simulink model "kurtosis"  (R2012b)
settings: Solver=ode45  StartTime=0.0  StopTime=3171  RelTol=1e-3
libraries: xbsIndex_r4 x3174, casper_library_flow_control x64, casper_library_misc x1, simulink_xsg_bridge x1
(part 1 of 24)
settings Model: Creator=sgowda  LastModifiedBy=sgowda

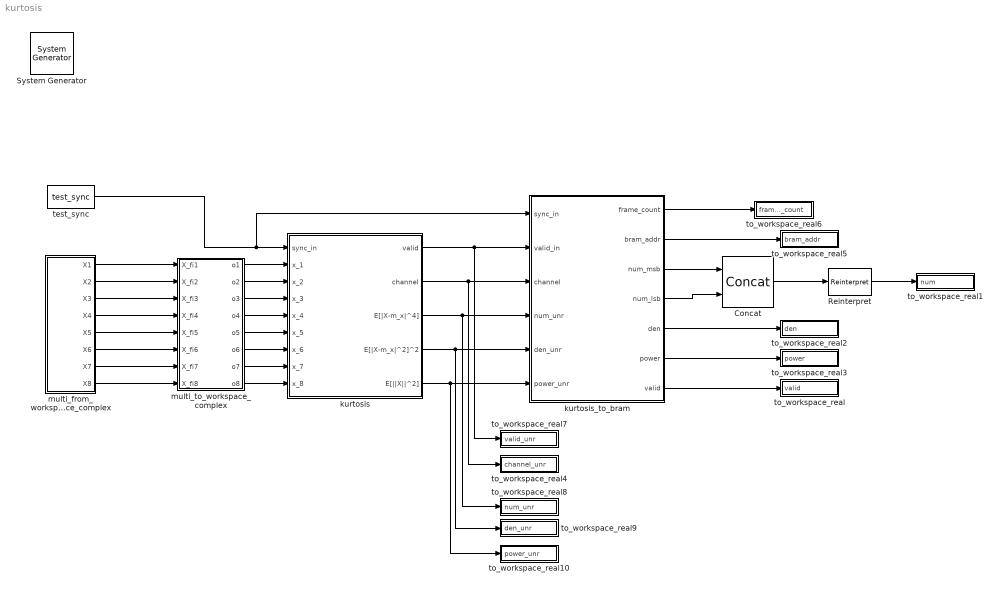
== system kurtosis ==
  " System Generator" : xbsIndex_r4/ System Generator  Tag=genX  xilinxfamily=Kintex7  part=xc7k325t  speed=-3  package=fbg676  synthesis_tool=XST  clock_wrapper=Clock Enables  directory=./netlist  proj_type=Project Navigator  Synth_file=XST Defaults  Impl_file=ISE Defaults  testbench=off  simulink_period=1  sysclk_period=10  dcm_input_clock_period=10  incr_netlist=off  trim_vbits=Everywhere in SubSystem  dbl_ovrd=According to Block Masks  core_generation=According to Block Masks  run_coregen=off  deprecated_control=off  eval_field=0  block_type=sysgen
  Concat : xbsIndex_r4/Concat  num_inputs=2  dbl_ovrd=off  block_type=concat
  Reinterpret : xbsIndex_r4/Reinterpret  force_arith_type=on  arith_type="Signed  (2's comp)"  force_bin_pt=on  bin_pt=84  block_type=reinterpret
  kurtosis : Subsystem
  kurtosis_to_bram : Subsystem
  multi_from_workspace_complex : Subsystem  mask{var_name=X, n_bits=18, bin_pt=17, quantization=Truncate, overflow=Wrap, arith_type=Signed  (2's comp), n_inputs=8}
      mask prompts: var_name "Workspace variable name"; n_bits "# of bits"; bin_pt "Binary Point"; arith_type "Arithmetic type"; n_inputs "# of inputs"
      mask init:
      | config.source = str2func('multi_mat_input_data_cplx_init_xblock');
      |  config.toplevel = gcb();
      |  xBlock(config, {config.toplevel, 'var_name', var_name, ...
      |      'n_bits', n_bits, 'bin_pt', bin_pt, 'quantization', quantization, ...
      |      'overflow', overflow, 'arith_type', arith_type, 'n_inputs', n_inputs});
      mask TypeOptions quantization: Truncate | Round  (unbiased: +/- Inf) | Round  (unbiased: Even Values)
      mask TypeOptions overflow: Wrap | Saturate | Flag as error
      mask TypeOptions arith_type: Signed  (2's comp) | Boolean | Unsigned
  multi_to_workspace_complex : Subsystem  mask{var_name=X_fi, n_bits=18, bin_pt=17, n_inputs=8}
      mask prompts: var_name "Workspace variable name"; n_bits "# of bits"; bin_pt "Binary Point"; n_inputs "# of inputs"
      mask init:
      | config.source = str2func('multi_mat_output_data_cplx_init_xblock');
      | config.toplevel = gcb();
      | xBlock(config, {config.toplevel, 'var_name', var_name, ...
      |     'n_bits', n_bits, 'bin_pt', bin_pt, 'n_inputs', n_inputs});
  test_sync : simulink_xsg_bridge/test_sync
  to_workspace_real : Subsystem  mask{var_name=valid}
      mask prompts: var_name "Workspace variable name"
      mask init:
      | config.source = str2func('mat_output_data_init_xblock');
      | config.toplevel = gcb();
      | xBlock(config, {config.toplevel, 'var_name', var_name});
  to_workspace_real1 : Subsystem  mask{var_name=num}
      mask prompts: var_name "Workspace variable name"
      mask init:
      | config.source = str2func('mat_output_data_init_xblock');
      | config.toplevel = gcb();
      | xBlock(config, {config.toplevel, 'var_name', var_name});
  to_workspace_real10 : Subsystem  mask{var_name=power_unr}
      mask prompts: var_name "Workspace variable name"
      mask init:
      | config.source = str2func('mat_output_data_init_xblock');
      | config.toplevel = gcb();
      | xBlock(config, {config.toplevel, 'var_name', var_name});
  to_workspace_real2 : Subsystem  mask{var_name=den}
      mask prompts: var_name "Workspace variable name"
      mask init:
      | config.source = str2func('mat_output_data_init_xblock');
      | config.toplevel = gcb();
      | xBlock(config, {config.toplevel, 'var_name', var_name});
  to_workspace_real3 : Subsystem  mask{var_name=power}
      mask prompts: var_name "Workspace variable name"
      mask init:
      | config.source = str2func('mat_output_data_init_xblock');
      | config.toplevel = gcb();
      | xBlock(config, {config.toplevel, 'var_name', var_name});
  to_workspace_real4 : Subsystem  mask{var_name=channel_unr}
      mask prompts: var_name "Workspace variable name"
      mask init:
      | config.source = str2func('mat_output_data_init_xblock');
      | config.toplevel = gcb();
      | xBlock(config, {config.toplevel, 'var_name', var_name});
  to_workspace_real5 : Subsystem  mask{var_name=bram_addr}
      mask prompts: var_name "Workspace variable name"
      mask init:
      | config.source = str2func('mat_output_data_init_xblock');
      | config.toplevel = gcb();
      | xBlock(config, {config.toplevel, 'var_name', var_name});
  to_workspace_real6 : Subsystem  mask{var_name=frame_count}
      mask prompts: var_name "Workspace variable name"
      mask init:
      | config.source = str2func('mat_output_data_init_xblock');
      | config.toplevel = gcb();
      | xBlock(config, {config.toplevel, 'var_name', var_name});
  to_workspace_real7 : Subsystem  mask{var_name=valid_unr}
      mask prompts: var_name "Workspace variable name"
      mask init:
      | config.source = str2func('mat_output_data_init_xblock');
      | config.toplevel = gcb();
      | xBlock(config, {config.toplevel, 'var_name', var_name});
  to_workspace_real8 : Subsystem  mask{var_name=num_unr}
      mask prompts: var_name "Workspace variable name"
      mask init:
      | config.source = str2func('mat_output_data_init_xblock');
      | config.toplevel = gcb();
      | xBlock(config, {config.toplevel, 'var_name', var_name});
  to_workspace_real9 : Subsystem  mask{var_name=den_unr}
      mask prompts: var_name "Workspace variable name"
      mask init:
      | config.source = str2func('mat_output_data_init_xblock');
      | config.toplevel = gcb();
      | xBlock(config, {config.toplevel, 'var_name', var_name});
  wires:
  test_sync/1 -> kurtosis_to_bram/1(sync_in), kurtosis/1(sync_in)
  multi_to_workspace_complex/2(o2) -> kurtosis/3(x_2)
  multi_to_workspace_complex/1(o1) -> kurtosis/2(x_1)
  multi_to_workspace_complex/6(o6) -> kurtosis/7(x_6)
  multi_to_workspace_complex/8(o8) -> kurtosis/9(x_8)
  multi_to_workspace_complex/7(o7) -> kurtosis/8(x_7)
  multi_to_workspace_complex/4(o4) -> kurtosis/5(x_4)
  multi_to_workspace_complex/3(o3) -> kurtosis/4(x_3)
  multi_to_workspace_complex/5(o5) -> kurtosis/6(x_5)
  multi_from_workspace_complex/1(X1) -> multi_to_workspace_complex/1(X_fi1)
  multi_from_workspace_complex/8(X8) -> multi_to_workspace_complex/8(X_fi8)
  multi_from_workspace_complex/2(X2) -> multi_to_workspace_complex/2(X_fi2)
  multi_from_workspace_complex/4(X4) -> multi_to_workspace_complex/4(X_fi4)
  multi_from_workspace_complex/7(X7) -> multi_to_workspace_complex/7(X_fi7)
  multi_from_workspace_complex/3(X3) -> multi_to_workspace_complex/3(X_fi3)
  multi_from_workspace_complex/5(X5) -> multi_to_workspace_complex/5(X_fi5)
  multi_from_workspace_complex/6(X6) -> multi_to_workspace_complex/6(X_fi6)
  kurtosis/1(valid) -> to_workspace_real7/1(valid_unr), kurtosis_to_bram/2(valid_in)
  kurtosis/2(channel) -> to_workspace_real4/1(channel_unr), kurtosis_to_bram/3(channel)
  kurtosis/3(E[|X-m_x|^4]) -> kurtosis_to_bram/4(num_unr), to_workspace_real8/1(num_unr)
  kurtosis/4(E[|X-m_x|^2]^2) -> to_workspace_real9/1(den_unr), kurtosis_to_bram/5(den_unr)
  kurtosis_to_bram/1(frame_count) -> to_workspace_real6/1(frame_count)
  kurtosis_to_bram/2(bram_addr) -> to_workspace_real5/1(bram_addr)
  kurtosis_to_bram/7(valid) -> to_workspace_real/1(valid)
  kurtosis_to_bram/5(den) -> to_workspace_real2/1(den)
  kurtosis_to_bram/6(power) -> to_workspace_real3/1(power)
  Reinterpret/1 -> to_workspace_real1/1(num)
  Concat/1 -> Reinterpret/1
  kurtosis_to_bram/3(num_msb) -> Concat/1
  kurtosis_to_bram/4(num_lsb) -> Concat/2
  kurtosis/5(E[||X||^2]) -> to_workspace_real10/1(power_unr), kurtosis_to_bram/6(power_unr)

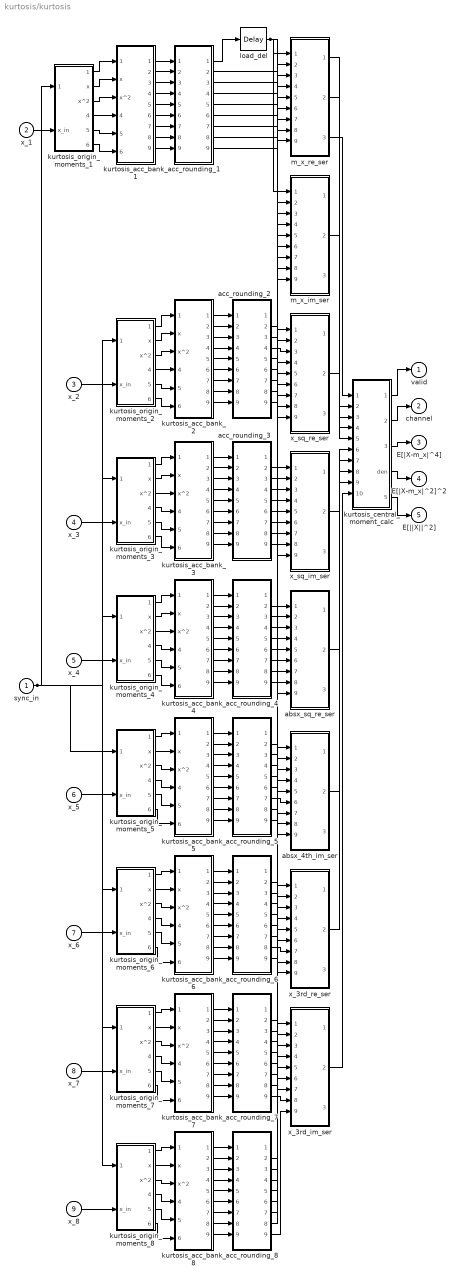
== system kurtosis/kurtosis ==
  sync_in : Inport
  x_1 : Inport  Port=2
  x_2 : Inport  Port=3
  x_3 : Inport  Port=4
  x_4 : Inport  Port=5
  x_5 : Inport  Port=6
  x_6 : Inport  Port=7
  x_7 : Inport  Port=8
  x_8 : Inport  Port=9
  absx_4th_im_ser : Subsystem
  absx_sq_re_ser : Subsystem
  acc_rounding_1 : Subsystem
  acc_rounding_2 : Subsystem
  acc_rounding_3 : Subsystem
  acc_rounding_4 : Subsystem
  acc_rounding_5 : Subsystem
  acc_rounding_6 : Subsystem
  acc_rounding_7 : Subsystem
  acc_rounding_8 : Subsystem
  kurtosis_acc_bank_1 : Subsystem
  kurtosis_acc_bank_2 : Subsystem
  kurtosis_acc_bank_3 : Subsystem
  kurtosis_acc_bank_4 : Subsystem
  kurtosis_acc_bank_5 : Subsystem
  kurtosis_acc_bank_6 : Subsystem
  kurtosis_acc_bank_7 : Subsystem
  kurtosis_acc_bank_8 : Subsystem
  kurtosis_central_moment_calc : Subsystem
  kurtosis_origin_moments_1 : Subsystem
  kurtosis_origin_moments_2 : Subsystem
  kurtosis_origin_moments_3 : Subsystem
  kurtosis_origin_moments_4 : Subsystem
  kurtosis_origin_moments_5 : Subsystem
  kurtosis_origin_moments_6 : Subsystem
  kurtosis_origin_moments_7 : Subsystem
  kurtosis_origin_moments_8 : Subsystem
  load_del : xbsIndex_r4/Delay  rst=off  infoeditControl=Selection of Reset will increase slice count due to use of real FFs and instead of SRLs  en=off  latency=1  dbl_ovrd=off  reg_retiming=off  block_type=delay
  m_x_im_ser : Subsystem
  m_x_re_ser : Subsystem
  x_3rd_im_ser : Subsystem
  x_3rd_re_ser : Subsystem
  x_sq_im_ser : Subsystem
  x_sq_re_ser : Subsystem
  valid : Outport
  channel : Outport  Port=2
  E[|X-m_x|^4] : Outport  Port=3
  E[|X-m_x|^2]^2 : Outport  Port=4
  E[||X||^2] : Outport  Port=5
  wires:
  sync_in/1 -> kurtosis_origin_moments_8/1(sync_in), kurtosis_origin_moments_7/1(sync_in), kurtosis_origin_moments_6/1(sync_in), kurtosis_origin_moments_5/1(sync_in), kurtosis_origin_moments_4/1(sync_in), kurtosis_origin_moments_3/1(sync_in), kurtosis_origin_moments_2/1(sync_in), kurtosis_origin_moments_1/1(sync_in)
  load_del/1 -> x_3rd_im_ser/1(load), x_3rd_re_ser/1(load), absx_4th_im_ser/1(load), absx_sq_re_ser/1(load), x_sq_im_ser/1(load), x_sq_re_ser/1(load), m_x_im_ser/1(load), m_x_re_ser/1(load)
  kurtosis_central_moment_calc/5(power) -> E[||X||^2]/1
  kurtosis_central_moment_calc/4(den) -> E[|X-m_x|^2]^2/1
  kurtosis_central_moment_calc/3(num) -> E[|X-m_x|^4]/1
  kurtosis_central_moment_calc/2(channel) -> channel/1
  kurtosis_central_moment_calc/1(sync_out) -> valid/1
  x_3rd_im_ser/2(ser_data) -> kurtosis_central_moment_calc/10("Im{E[|X|^2X]}")
  x_3rd_re_ser/2(ser_data) -> kurtosis_central_moment_calc/9("Re{E[|X|^2X]}")
  absx_4th_im_ser/2(ser_data) -> kurtosis_central_moment_calc/8(E[||X||^4])
  absx_sq_re_ser/2(ser_data) -> kurtosis_central_moment_calc/7(E[|X|^2])
  x_sq_im_ser/2(ser_data) -> kurtosis_central_moment_calc/6("Im{E[X^2]}")
  x_sq_re_ser/2(ser_data) -> kurtosis_central_moment_calc/5("Re{E[X^2]}")
  m_x_im_ser/2(ser_data) -> kurtosis_central_moment_calc/4("Im{E[X]}")
  m_x_re_ser/2(ser_data) -> kurtosis_central_moment_calc/3("Re{E[X]}")
  m_x_re_ser/1(addr) -> kurtosis_central_moment_calc/2(channel_in)
  m_x_re_ser/3(valid) -> kurtosis_central_moment_calc/1(sync)
  acc_rounding_8/9(X_3rd_acc_im_rounded) -> x_3rd_im_ser/9(din_8)
  acc_rounding_7/9(X_3rd_acc_im_rounded) -> x_3rd_im_ser/8(din_7)
  acc_rounding_6/9(X_3rd_acc_im_rounded) -> x_3rd_im_ser/7(din_6)
  acc_rounding_5/9(X_3rd_acc_im_rounded) -> x_3rd_im_ser/6(din_5)
  acc_rounding_4/9(X_3rd_acc_im_rounded) -> x_3rd_im_ser/5(din_4)
  acc_rounding_3/9(X_3rd_acc_im_rounded) -> x_3rd_im_ser/4(din_3)
  acc_rounding_2/9(X_3rd_acc_im_rounded) -> x_3rd_im_ser/3(din_2)
  acc_rounding_1/9(X_3rd_acc_im_rounded) -> x_3rd_im_ser/2(din_1)
  acc_rounding_8/8(X_3rd_acc_re_rounded) -> x_3rd_re_ser/9(din_8)
  acc_rounding_7/8(X_3rd_acc_re_rounded) -> x_3rd_re_ser/8(din_7)
  acc_rounding_6/8(X_3rd_acc_re_rounded) -> x_3rd_re_ser/7(din_6)
  acc_rounding_5/8(X_3rd_acc_re_rounded) -> x_3rd_re_ser/6(din_5)
  acc_rounding_4/8(X_3rd_acc_re_rounded) -> x_3rd_re_ser/5(din_4)
  acc_rounding_3/8(X_3rd_acc_re_rounded) -> x_3rd_re_ser/4(din_3)
  acc_rounding_2/8(X_3rd_acc_re_rounded) -> x_3rd_re_ser/3(din_2)
  acc_rounding_1/8(X_3rd_acc_re_rounded) -> x_3rd_re_ser/2(din_1)
  acc_rounding_8/7(abs_X_4th_rounded) -> absx_4th_im_ser/9(din_8)
  acc_rounding_7/7(abs_X_4th_rounded) -> absx_4th_im_ser/8(din_7)
  acc_rounding_6/7(abs_X_4th_rounded) -> absx_4th_im_ser/7(din_6)
  acc_rounding_5/7(abs_X_4th_rounded) -> absx_4th_im_ser/6(din_5)
  acc_rounding_4/7(abs_X_4th_rounded) -> absx_4th_im_ser/5(din_4)
  acc_rounding_3/7(abs_X_4th_rounded) -> absx_4th_im_ser/4(din_3)
  acc_rounding_2/7(abs_X_4th_rounded) -> absx_4th_im_ser/3(din_2)
  acc_rounding_1/7(abs_X_4th_rounded) -> absx_4th_im_ser/2(din_1)
  acc_rounding_8/6(abs_X_sq_acc_rounded) -> absx_sq_re_ser/9(din_8)
  acc_rounding_7/6(abs_X_sq_acc_rounded) -> absx_sq_re_ser/8(din_7)
  acc_rounding_6/6(abs_X_sq_acc_rounded) -> absx_sq_re_ser/7(din_6)
  acc_rounding_5/6(abs_X_sq_acc_rounded) -> absx_sq_re_ser/6(din_5)
  acc_rounding_4/6(abs_X_sq_acc_rounded) -> absx_sq_re_ser/5(din_4)
  acc_rounding_3/6(abs_X_sq_acc_rounded) -> absx_sq_re_ser/4(din_3)
  acc_rounding_2/6(abs_X_sq_acc_rounded) -> absx_sq_re_ser/3(din_2)
  acc_rounding_1/6(abs_X_sq_acc_rounded) -> absx_sq_re_ser/2(din_1)
  acc_rounding_8/5(X_sq_acc_im_rounded) -> x_sq_im_ser/9(din_8)
  acc_rounding_7/5(X_sq_acc_im_rounded) -> x_sq_im_ser/8(din_7)
  acc_rounding_6/5(X_sq_acc_im_rounded) -> x_sq_im_ser/7(din_6)
  acc_rounding_5/5(X_sq_acc_im_rounded) -> x_sq_im_ser/6(din_5)
  acc_rounding_4/5(X_sq_acc_im_rounded) -> x_sq_im_ser/5(din_4)
  acc_rounding_3/5(X_sq_acc_im_rounded) -> x_sq_im_ser/4(din_3)
  acc_rounding_2/5(X_sq_acc_im_rounded) -> x_sq_im_ser/3(din_2)
  acc_rounding_1/5(X_sq_acc_im_rounded) -> x_sq_im_ser/2(din_1)
  acc_rounding_8/4(X_sq_acc_re_rounded) -> x_sq_re_ser/9(din_8)
  acc_rounding_7/4(X_sq_acc_re_rounded) -> x_sq_re_ser/8(din_7)
  acc_rounding_6/4(X_sq_acc_re_rounded) -> x_sq_re_ser/7(din_6)
  acc_rounding_5/4(X_sq_acc_re_rounded) -> x_sq_re_ser/6(din_5)
  acc_rounding_4/4(X_sq_acc_re_rounded) -> x_sq_re_ser/5(din_4)
  acc_rounding_3/4(X_sq_acc_re_rounded) -> x_sq_re_ser/4(din_3)
  acc_rounding_2/4(X_sq_acc_re_rounded) -> x_sq_re_ser/3(din_2)
  acc_rounding_1/4(X_sq_acc_re_rounded) -> x_sq_re_ser/2(din_1)
  acc_rounding_8/3(m_x_im_rounded) -> m_x_im_ser/9(din_8)
  acc_rounding_7/3(m_x_im_rounded) -> m_x_im_ser/8(din_7)
  acc_rounding_6/3(m_x_im_rounded) -> m_x_im_ser/7(din_6)
  acc_rounding_5/3(m_x_im_rounded) -> m_x_im_ser/6(din_5)
  acc_rounding_4/3(m_x_im_rounded) -> m_x_im_ser/5(din_4)
  acc_rounding_3/3(m_x_im_rounded) -> m_x_im_ser/4(din_3)
  acc_rounding_2/3(m_x_im_rounded) -> m_x_im_ser/3(din_2)
  acc_rounding_1/3(m_x_im_rounded) -> m_x_im_ser/2(din_1)
  acc_rounding_8/2(m_x_re_rounded) -> m_x_re_ser/9(din_8)
  acc_rounding_7/2(m_x_re_rounded) -> m_x_re_ser/8(din_7)
  acc_rounding_6/2(m_x_re_rounded) -> m_x_re_ser/7(din_6)
  acc_rounding_5/2(m_x_re_rounded) -> m_x_re_ser/6(din_5)
  acc_rounding_4/2(m_x_re_rounded) -> m_x_re_ser/5(din_4)
  acc_rounding_3/2(m_x_re_rounded) -> m_x_re_ser/4(din_3)
  acc_rounding_2/2(m_x_re_rounded) -> m_x_re_ser/3(din_2)
  acc_rounding_1/2(m_x_re_rounded) -> m_x_re_ser/2(din_1)
  acc_rounding_1/1(sync_out) -> load_del/1
  kurtosis_acc_bank_8/9("Im{E[x|x|^2]}") -> acc_rounding_8/9(X_3rd_acc_im)
  kurtosis_acc_bank_8/8("Re{E[x|x|^2]}") -> acc_rounding_8/8(X_3rd_acc_re)
  kurtosis_acc_bank_8/7(E[|x|^4]) -> acc_rounding_8/7(abs_X_4th_acc)
  kurtosis_acc_bank_8/6(E[|x|^2]) -> acc_rounding_8/6(abs_X_sq_acc)
  kurtosis_acc_bank_8/5("Im{E[x^2]}") -> acc_rounding_8/5(X_sq_acc_im)
  kurtosis_acc_bank_8/4("Re{E[x^2]}") -> acc_rounding_8/4(X_sq_acc_re)
  kurtosis_acc_bank_8/3("Im{E[x]}") -> acc_rounding_8/3(x_acc_im)
  kurtosis_acc_bank_8/2("Re{E[x]}") -> acc_rounding_8/2(x_acc_re)
  kurtosis_acc_bank_8/1(sync_out) -> acc_rounding_8/1(sync)
  kurtosis_origin_moments_8/6(x|x|^2) -> kurtosis_acc_bank_8/6(x|x|^2)
  kurtosis_origin_moments_8/5(|x|^4) -> kurtosis_acc_bank_8/5(|x|^4)
  kurtosis_origin_moments_8/4(|x|^2) -> kurtosis_acc_bank_8/4(|x|^2)
  kurtosis_origin_moments_8/3(x^2) -> kurtosis_acc_bank_8/3(x^2)
  kurtosis_origin_moments_8/2(x) -> kurtosis_acc_bank_8/2(x)
  kurtosis_origin_moments_8/1(sync_out) -> kurtosis_acc_bank_8/1(sync)
  x_8/1 -> kurtosis_origin_moments_8/2(x_in)
  kurtosis_acc_bank_7/9("Im{E[x|x|^2]}") -> acc_rounding_7/9(X_3rd_acc_im)
  kurtosis_acc_bank_7/8("Re{E[x|x|^2]}") -> acc_rounding_7/8(X_3rd_acc_re)
  kurtosis_acc_bank_7/7(E[|x|^4]) -> acc_rounding_7/7(abs_X_4th_acc)
  kurtosis_acc_bank_7/6(E[|x|^2]) -> acc_rounding_7/6(abs_X_sq_acc)
  kurtosis_acc_bank_7/5("Im{E[x^2]}") -> acc_rounding_7/5(X_sq_acc_im)
  kurtosis_acc_bank_7/4("Re{E[x^2]}") -> acc_rounding_7/4(X_sq_acc_re)
  kurtosis_acc_bank_7/3("Im{E[x]}") -> acc_rounding_7/3(x_acc_im)
  kurtosis_acc_bank_7/2("Re{E[x]}") -> acc_rounding_7/2(x_acc_re)
  kurtosis_acc_bank_7/1(sync_out) -> acc_rounding_7/1(sync)
  kurtosis_origin_moments_7/6(x|x|^2) -> kurtosis_acc_bank_7/6(x|x|^2)
  kurtosis_origin_moments_7/5(|x|^4) -> kurtosis_acc_bank_7/5(|x|^4)
  kurtosis_origin_moments_7/4(|x|^2) -> kurtosis_acc_bank_7/4(|x|^2)
  kurtosis_origin_moments_7/3(x^2) -> kurtosis_acc_bank_7/3(x^2)
  kurtosis_origin_moments_7/2(x) -> kurtosis_acc_bank_7/2(x)
  kurtosis_origin_moments_7/1(sync_out) -> kurtosis_acc_bank_7/1(sync)
  x_7/1 -> kurtosis_origin_moments_7/2(x_in)
  kurtosis_acc_bank_6/9("Im{E[x|x|^2]}") -> acc_rounding_6/9(X_3rd_acc_im)
  kurtosis_acc_bank_6/8("Re{E[x|x|^2]}") -> acc_rounding_6/8(X_3rd_acc_re)
  kurtosis_acc_bank_6/7(E[|x|^4]) -> acc_rounding_6/7(abs_X_4th_acc)
  kurtosis_acc_bank_6/6(E[|x|^2]) -> acc_rounding_6/6(abs_X_sq_acc)
  kurtosis_acc_bank_6/5("Im{E[x^2]}") -> acc_rounding_6/5(X_sq_acc_im)
  kurtosis_acc_bank_6/4("Re{E[x^2]}") -> acc_rounding_6/4(X_sq_acc_re)
  kurtosis_acc_bank_6/3("Im{E[x]}") -> acc_rounding_6/3(x_acc_im)
  kurtosis_acc_bank_6/2("Re{E[x]}") -> acc_rounding_6/2(x_acc_re)
  kurtosis_acc_bank_6/1(sync_out) -> acc_rounding_6/1(sync)
  kurtosis_origin_moments_6/6(x|x|^2) -> kurtosis_acc_bank_6/6(x|x|^2)
  kurtosis_origin_moments_6/5(|x|^4) -> kurtosis_acc_bank_6/5(|x|^4)
  kurtosis_origin_moments_6/4(|x|^2) -> kurtosis_acc_bank_6/4(|x|^2)
  kurtosis_origin_moments_6/3(x^2) -> kurtosis_acc_bank_6/3(x^2)
  kurtosis_origin_moments_6/2(x) -> kurtosis_acc_bank_6/2(x)
  kurtosis_origin_moments_6/1(sync_out) -> kurtosis_acc_bank_6/1(sync)
  x_6/1 -> kurtosis_origin_moments_6/2(x_in)
  kurtosis_acc_bank_5/9("Im{E[x|x|^2]}") -> acc_rounding_5/9(X_3rd_acc_im)
  kurtosis_acc_bank_5/8("Re{E[x|x|^2]}") -> acc_rounding_5/8(X_3rd_acc_re)
  kurtosis_acc_bank_5/7(E[|x|^4]) -> acc_rounding_5/7(abs_X_4th_acc)
  kurtosis_acc_bank_5/6(E[|x|^2]) -> acc_rounding_5/6(abs_X_sq_acc)
  kurtosis_acc_bank_5/5("Im{E[x^2]}") -> acc_rounding_5/5(X_sq_acc_im)
  kurtosis_acc_bank_5/4("Re{E[x^2]}") -> acc_rounding_5/4(X_sq_acc_re)
  kurtosis_acc_bank_5/3("Im{E[x]}") -> acc_rounding_5/3(x_acc_im)
  kurtosis_acc_bank_5/2("Re{E[x]}") -> acc_rounding_5/2(x_acc_re)
  kurtosis_acc_bank_5/1(sync_out) -> acc_rounding_5/1(sync)
  kurtosis_origin_moments_5/6(x|x|^2) -> kurtosis_acc_bank_5/6(x|x|^2)
  kurtosis_origin_moments_5/5(|x|^4) -> kurtosis_acc_bank_5/5(|x|^4)
  kurtosis_origin_moments_5/4(|x|^2) -> kurtosis_acc_bank_5/4(|x|^2)
  kurtosis_origin_moments_5/3(x^2) -> kurtosis_acc_bank_5/3(x^2)
  kurtosis_origin_moments_5/2(x) -> kurtosis_acc_bank_5/2(x)
  kurtosis_origin_moments_5/1(sync_out) -> kurtosis_acc_bank_5/1(sync)
  x_5/1 -> kurtosis_origin_moments_5/2(x_in)
  kurtosis_acc_bank_4/9("Im{E[x|x|^2]}") -> acc_rounding_4/9(X_3rd_acc_im)
  kurtosis_acc_bank_4/8("Re{E[x|x|^2]}") -> acc_rounding_4/8(X_3rd_acc_re)
  kurtosis_acc_bank_4/7(E[|x|^4]) -> acc_rounding_4/7(abs_X_4th_acc)
  kurtosis_acc_bank_4/6(E[|x|^2]) -> acc_rounding_4/6(abs_X_sq_acc)
  kurtosis_acc_bank_4/5("Im{E[x^2]}") -> acc_rounding_4/5(X_sq_acc_im)
  kurtosis_acc_bank_4/4("Re{E[x^2]}") -> acc_rounding_4/4(X_sq_acc_re)
  kurtosis_acc_bank_4/3("Im{E[x]}") -> acc_rounding_4/3(x_acc_im)
  kurtosis_acc_bank_4/2("Re{E[x]}") -> acc_rounding_4/2(x_acc_re)
  kurtosis_acc_bank_4/1(sync_out) -> acc_rounding_4/1(sync)
  kurtosis_origin_moments_4/6(x|x|^2) -> kurtosis_acc_bank_4/6(x|x|^2)
  kurtosis_origin_moments_4/5(|x|^4) -> kurtosis_acc_bank_4/5(|x|^4)
  kurtosis_origin_moments_4/4(|x|^2) -> kurtosis_acc_bank_4/4(|x|^2)
  kurtosis_origin_moments_4/3(x^2) -> kurtosis_acc_bank_4/3(x^2)
  kurtosis_origin_moments_4/2(x) -> kurtosis_acc_bank_4/2(x)
  kurtosis_origin_moments_4/1(sync_out) -> kurtosis_acc_bank_4/1(sync)
  x_4/1 -> kurtosis_origin_moments_4/2(x_in)
  kurtosis_acc_bank_3/9("Im{E[x|x|^2]}") -> acc_rounding_3/9(X_3rd_acc_im)
  kurtosis_acc_bank_3/8("Re{E[x|x|^2]}") -> acc_rounding_3/8(X_3rd_acc_re)
  kurtosis_acc_bank_3/7(E[|x|^4]) -> acc_rounding_3/7(abs_X_4th_acc)
  kurtosis_acc_bank_3/6(E[|x|^2]) -> acc_rounding_3/6(abs_X_sq_acc)
  kurtosis_acc_bank_3/5("Im{E[x^2]}") -> acc_rounding_3/5(X_sq_acc_im)
  kurtosis_acc_bank_3/4("Re{E[x^2]}") -> acc_rounding_3/4(X_sq_acc_re)
  kurtosis_acc_bank_3/3("Im{E[x]}") -> acc_rounding_3/3(x_acc_im)
  kurtosis_acc_bank_3/2("Re{E[x]}") -> acc_rounding_3/2(x_acc_re)
  kurtosis_acc_bank_3/1(sync_out) -> acc_rounding_3/1(sync)
  kurtosis_origin_moments_3/6(x|x|^2) -> kurtosis_acc_bank_3/6(x|x|^2)
  kurtosis_origin_moments_3/5(|x|^4) -> kurtosis_acc_bank_3/5(|x|^4)
  kurtosis_origin_moments_3/4(|x|^2) -> kurtosis_acc_bank_3/4(|x|^2)
  kurtosis_origin_moments_3/3(x^2) -> kurtosis_acc_bank_3/3(x^2)
  kurtosis_origin_moments_3/2(x) -> kurtosis_acc_bank_3/2(x)
  kurtosis_origin_moments_3/1(sync_out) -> kurtosis_acc_bank_3/1(sync)
  x_3/1 -> kurtosis_origin_moments_3/2(x_in)
  kurtosis_acc_bank_2/9("Im{E[x|x|^2]}") -> acc_rounding_2/9(X_3rd_acc_im)
  kurtosis_acc_bank_2/8("Re{E[x|x|^2]}") -> acc_rounding_2/8(X_3rd_acc_re)
  kurtosis_acc_bank_2/7(E[|x|^4]) -> acc_rounding_2/7(abs_X_4th_acc)
  kurtosis_acc_bank_2/6(E[|x|^2]) -> acc_rounding_2/6(abs_X_sq_acc)
  kurtosis_acc_bank_2/5("Im{E[x^2]}") -> acc_rounding_2/5(X_sq_acc_im)
  kurtosis_acc_bank_2/4("Re{E[x^2]}") -> acc_rounding_2/4(X_sq_acc_re)
  kurtosis_acc_bank_2/3("Im{E[x]}") -> acc_rounding_2/3(x_acc_im)
  kurtosis_acc_bank_2/2("Re{E[x]}") -> acc_rounding_2/2(x_acc_re)
  kurtosis_acc_bank_2/1(sync_out) -> acc_rounding_2/1(sync)
  kurtosis_origin_moments_2/6(x|x|^2) -> kurtosis_acc_bank_2/6(x|x|^2)
  kurtosis_origin_moments_2/5(|x|^4) -> kurtosis_acc_bank_2/5(|x|^4)
  kurtosis_origin_moments_2/4(|x|^2) -> kurtosis_acc_bank_2/4(|x|^2)
  kurtosis_origin_moments_2/3(x^2) -> kurtosis_acc_bank_2/3(x^2)
  kurtosis_origin_moments_2/2(x) -> kurtosis_acc_bank_2/2(x)
  kurtosis_origin_moments_2/1(sync_out) -> kurtosis_acc_bank_2/1(sync)
  x_2/1 -> kurtosis_origin_moments_2/2(x_in)
  kurtosis_acc_bank_1/9("Im{E[x|x|^2]}") -> acc_rounding_1/9(X_3rd_acc_im)
  kurtosis_acc_bank_1/8("Re{E[x|x|^2]}") -> acc_rounding_1/8(X_3rd_acc_re)
  kurtosis_acc_bank_1/7(E[|x|^4]) -> acc_rounding_1/7(abs_X_4th_acc)
  kurtosis_acc_bank_1/6(E[|x|^2]) -> acc_rounding_1/6(abs_X_sq_acc)
  kurtosis_acc_bank_1/5("Im{E[x^2]}") -> acc_rounding_1/5(X_sq_acc_im)
  kurtosis_acc_bank_1/4("Re{E[x^2]}") -> acc_rounding_1/4(X_sq_acc_re)
  kurtosis_acc_bank_1/3("Im{E[x]}") -> acc_rounding_1/3(x_acc_im)
  kurtosis_acc_bank_1/2("Re{E[x]}") -> acc_rounding_1/2(x_acc_re)
  kurtosis_acc_bank_1/1(sync_out) -> acc_rounding_1/1(sync)
  kurtosis_origin_moments_1/6(x|x|^2) -> kurtosis_acc_bank_1/6(x|x|^2)
  kurtosis_origin_moments_1/5(|x|^4) -> kurtosis_acc_bank_1/5(|x|^4)
  kurtosis_origin_moments_1/4(|x|^2) -> kurtosis_acc_bank_1/4(|x|^2)
  kurtosis_origin_moments_1/3(x^2) -> kurtosis_acc_bank_1/3(x^2)
  kurtosis_origin_moments_1/2(x) -> kurtosis_acc_bank_1/2(x)
  kurtosis_origin_moments_1/1(sync_out) -> kurtosis_acc_bank_1/1(sync)
  x_1/1 -> kurtosis_origin_moments_1/2(x_in)

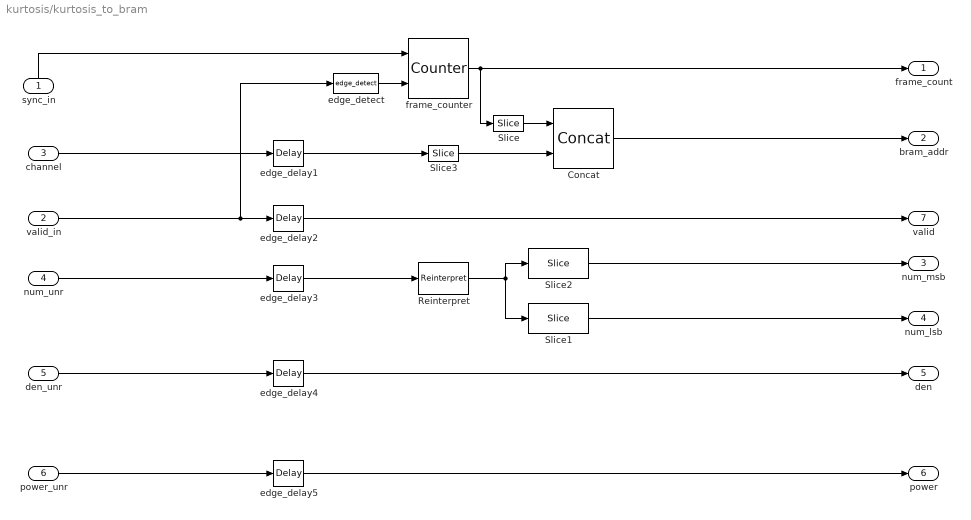
== system kurtosis/kurtosis_to_bram ==
  sync_in : Inport
  valid_in : Inport  Port=2
  channel : Inport  Port=3
  num_unr : Inport  Port=4
  den_unr : Inport  Port=5
  power_unr : Inport  Port=6
  Concat : xbsIndex_r4/Concat  num_inputs=2  dbl_ovrd=off  block_type=concat
  Reinterpret : xbsIndex_r4/Reinterpret  force_arith_type=on  arith_type=Unsigned  force_bin_pt=on  bin_pt=0  block_type=reinterpret
  Slice : xbsIndex_r4/Slice  nbits=7  boolean_output=off  mode=Lower Bit Location + Width  bit1=0  base1=MSB of Input  bit0=0  base0=LSB of Input  dbl_ovrd=off  block_type=slice
  Slice1 : xbsIndex_r4/Slice  nbits=64  boolean_output=off  mode=Lower Bit Location + Width  bit1=0  base1=MSB of Input  bit0=0  base0=LSB of Input  dbl_ovrd=off  block_type=slice
  Slice2 : xbsIndex_r4/Slice  nbits=32  boolean_output=off  mode=Lower Bit Location + Width  bit1=0  base1=MSB of Input  bit0=64  base0=LSB of Input  dbl_ovrd=off  block_type=slice
  Slice3 : xbsIndex_r4/Slice  nbits=3  boolean_output=off  mode=Lower Bit Location + Width  bit1=0  base1=MSB of Input  bit0=0  base0=LSB of Input  dbl_ovrd=off  block_type=slice
  edge_delay{1..5} (5 alike) : xbsIndex_r4/Delay  rst=off  infoeditControl=Selection of Reset will increase slice count due to use of real FFs and instead of SRLs  en=off  latency=1  dbl_ovrd=off  reg_retiming=off  block_type=delay
  edge_detect : casper_library_misc/edge_detect  edge=Rising  polarity=Active High  x_in=[0 0.08 0.08 0.16 0.16 0.24 0.24 0.32 0.32 0.4]  y_in="[-1 -1  1  1  1  1  1  1  1  1]"  x_out=[0.6 0.68 0.68 0.76 0.76 0.84 0.84 0.92 0.92 1]  y_out="[-1 -1  1  1 -1 -1 -1 -1 -1 -1]"
  frame_counter : xbsIndex_r4/Counter  cnt_type=Free Running  cnt_to=Inf  operation=Up  start_count=0  cnt_by_val=1  arith_type=Unsigned  n_bits=48  bin_pt=0  load_pin=off  rst=on  en=on  explicit_period=on  period=1  dbl_ovrd=off  use_behavioral_HDL=off  implementation=DSP48  block_type=counter
  frame_count : Outport
  bram_addr : Outport  Port=2
  num_msb : Outport  Port=3
  num_lsb : Outport  Port=4
  den : Outport  Port=5
  power : Outport  Port=6
  valid : Outport  Port=7
  wires:
  Slice3/1 -> Concat/2
  Slice/1 -> Concat/1
  valid_in/1 -> edge_detect/1, edge_delay2/1
  edge_delay1/1 -> Slice3/1
  Concat/1 -> bram_addr/1
  edge_detect/1 -> frame_counter/2
  edge_delay5/1 -> power/1
  edge_delay4/1 -> den/1
  edge_delay3/1 -> Reinterpret/1
  frame_counter/1 -> frame_count/1, Slice/1
  channel/1 -> edge_delay1/1
  edge_delay2/1 -> valid/1
  Reinterpret/1 -> Slice1/1, Slice2/1
  sync_in/1 -> frame_counter/1
  Slice2/1 -> num_msb/1
  Slice1/1 -> num_lsb/1
  num_unr/1 -> edge_delay3/1
  den_unr/1 -> edge_delay4/1
  power_unr/1 -> edge_delay5/1

== system kurtosis/multi_from_workspace_complex ==
  from_workspace_cplx_1 : Subsystem
  from_workspace_cplx_2 : Subsystem
  from_workspace_cplx_3 : Subsystem
  from_workspace_cplx_4 : Subsystem
  from_workspace_cplx_5 : Subsystem
  from_workspace_cplx_6 : Subsystem
  from_workspace_cplx_7 : Subsystem
  from_workspace_cplx_8 : Subsystem
  X1 : Outport
  X2 : Outport  Port=2
  X3 : Outport  Port=3
  X4 : Outport  Port=4
  X5 : Outport  Port=5
  X6 : Outport  Port=6
  X7 : Outport  Port=7
  X8 : Outport  Port=8
  wires:
  from_workspace_cplx_8/1(X8) -> X8/1
  from_workspace_cplx_7/1(X7) -> X7/1
  from_workspace_cplx_6/1(X6) -> X6/1
  from_workspace_cplx_5/1(X5) -> X5/1
  from_workspace_cplx_4/1(X4) -> X4/1
  from_workspace_cplx_3/1(X3) -> X3/1
  from_workspace_cplx_2/1(X2) -> X2/1
  from_workspace_cplx_1/1(X1) -> X1/1

== system kurtosis/multi_to_workspace_complex ==
  X_fi1 : Inport
  X_fi2 : Inport  Port=2
  X_fi3 : Inport  Port=3
  X_fi4 : Inport  Port=4
  X_fi5 : Inport  Port=5
  X_fi6 : Inport  Port=6
  X_fi7 : Inport  Port=7
  X_fi8 : Inport  Port=8
  to_workspace_cplx_1 : Subsystem
  to_workspace_cplx_2 : Subsystem
  to_workspace_cplx_3 : Subsystem
  to_workspace_cplx_4 : Subsystem
  to_workspace_cplx_5 : Subsystem
  to_workspace_cplx_6 : Subsystem
  to_workspace_cplx_7 : Subsystem
  to_workspace_cplx_8 : Subsystem
  o1 : Outport
  o2 : Outport  Port=2
  o3 : Outport  Port=3
  o4 : Outport  Port=4
  o5 : Outport  Port=5
  o6 : Outport  Port=6
  o7 : Outport  Port=7
  o8 : Outport  Port=8
  wires:
  to_workspace_cplx_8/1(_o) -> o8/1
  X_fi8/1 -> to_workspace_cplx_8/1(X_fi8)
  to_workspace_cplx_7/1(_o) -> o7/1
  X_fi7/1 -> to_workspace_cplx_7/1(X_fi7)
  to_workspace_cplx_6/1(_o) -> o6/1
  X_fi6/1 -> to_workspace_cplx_6/1(X_fi6)
  to_workspace_cplx_5/1(_o) -> o5/1
  X_fi5/1 -> to_workspace_cplx_5/1(X_fi5)
  to_workspace_cplx_4/1(_o) -> o4/1
  X_fi4/1 -> to_workspace_cplx_4/1(X_fi4)
  to_workspace_cplx_3/1(_o) -> o3/1
  X_fi3/1 -> to_workspace_cplx_3/1(X_fi3)
  to_workspace_cplx_2/1(_o) -> o2/1
  X_fi2/1 -> to_workspace_cplx_2/1(X_fi2)
  to_workspace_cplx_1/1(_o) -> o1/1
  X_fi1/1 -> to_workspace_cplx_1/1(X_fi1)

== system kurtosis/to_workspace_real ==
  valid : Inport
  gateway : xbsIndex_r4/Gateway Out  inherit_from_input=on  hdl_port=off  timing_constraint=None  locs_specified=off  LOCs={}  UseAsDAC=off  DACChannel='1'  block_type=gatewayout
  workspace_input : ToWorkspace  VariableName=valid  SampleTime=-1
  wires:
  gateway/1 -> workspace_input/1
  valid/1 -> gateway/1

== system kurtosis/to_workspace_real1 ==
  num : Inport
  gateway : xbsIndex_r4/Gateway Out  inherit_from_input=on  hdl_port=off  timing_constraint=None  locs_specified=off  LOCs={}  UseAsDAC=off  DACChannel='1'  block_type=gatewayout
  workspace_input : ToWorkspace  VariableName=num  SampleTime=-1
  wires:
  gateway/1 -> workspace_input/1
  num/1 -> gateway/1

== system kurtosis/to_workspace_real10 ==
  power_unr : Inport
  gateway : xbsIndex_r4/Gateway Out  inherit_from_input=on  hdl_port=off  timing_constraint=None  locs_specified=off  LOCs={}  UseAsDAC=off  DACChannel='1'  block_type=gatewayout
  workspace_input : ToWorkspace  VariableName=power_unr  SampleTime=-1
  wires:
  gateway/1 -> workspace_input/1
  power_unr/1 -> gateway/1

== system kurtosis/to_workspace_real2 ==
  den : Inport
  gateway : xbsIndex_r4/Gateway Out  inherit_from_input=on  hdl_port=off  timing_constraint=None  locs_specified=off  LOCs={}  UseAsDAC=off  DACChannel='1'  block_type=gatewayout
  workspace_input : ToWorkspace  VariableName=den  SampleTime=-1
  wires:
  gateway/1 -> workspace_input/1
  den/1 -> gateway/1

== system kurtosis/to_workspace_real3 ==
  power : Inport
  gateway : xbsIndex_r4/Gateway Out  inherit_from_input=on  hdl_port=off  timing_constraint=None  locs_specified=off  LOCs={}  UseAsDAC=off  DACChannel='1'  block_type=gatewayout
  workspace_input : ToWorkspace  VariableName=power  SampleTime=-1
  wires:
  gateway/1 -> workspace_input/1
  power/1 -> gateway/1

== system kurtosis/to_workspace_real4 ==
  channel_unr : Inport
  gateway : xbsIndex_r4/Gateway Out  inherit_from_input=on  hdl_port=off  timing_constraint=None  locs_specified=off  LOCs={}  UseAsDAC=off  DACChannel='1'  block_type=gatewayout
  workspace_input : ToWorkspace  VariableName=channel_unr  SampleTime=-1
  wires:
  gateway/1 -> workspace_input/1
  channel_unr/1 -> gateway/1

== system kurtosis/to_workspace_real5 ==
  bram_addr : Inport
  gateway : xbsIndex_r4/Gateway Out  inherit_from_input=on  hdl_port=off  timing_constraint=None  locs_specified=off  LOCs={}  UseAsDAC=off  DACChannel='1'  block_type=gatewayout
  workspace_input : ToWorkspace  VariableName=bram_addr  SampleTime=-1
  wires:
  gateway/1 -> workspace_input/1
  bram_addr/1 -> gateway/1

== system kurtosis/to_workspace_real6 ==
  frame_count : Inport
  gateway : xbsIndex_r4/Gateway Out  inherit_from_input=on  hdl_port=off  timing_constraint=None  locs_specified=off  LOCs={}  UseAsDAC=off  DACChannel='1'  block_type=gatewayout
  workspace_input : ToWorkspace  VariableName=frame_count  SampleTime=-1
  wires:
  gateway/1 -> workspace_input/1
  frame_count/1 -> gateway/1

== system kurtosis/to_workspace_real7 ==
  valid_unr : Inport
  gateway : xbsIndex_r4/Gateway Out  inherit_from_input=on  hdl_port=off  timing_constraint=None  locs_specified=off  LOCs={}  UseAsDAC=off  DACChannel='1'  block_type=gatewayout
  workspace_input : ToWorkspace  VariableName=valid_unr  SampleTime=-1
  wires:
  gateway/1 -> workspace_input/1
  valid_unr/1 -> gateway/1

== system kurtosis/to_workspace_real8 ==
  num_unr : Inport
  gateway : xbsIndex_r4/Gateway Out  inherit_from_input=on  hdl_port=off  timing_constraint=None  locs_specified=off  LOCs={}  UseAsDAC=off  DACChannel='1'  block_type=gatewayout
  workspace_input : ToWorkspace  VariableName=num_unr  SampleTime=-1
  wires:
  gateway/1 -> workspace_input/1
  num_unr/1 -> gateway/1

== system kurtosis/to_workspace_real9 ==
  den_unr : Inport
  gateway : xbsIndex_r4/Gateway Out  inherit_from_input=on  hdl_port=off  timing_constraint=None  locs_specified=off  LOCs={}  UseAsDAC=off  DACChannel='1'  block_type=gatewayout
  workspace_input : ToWorkspace  VariableName=den_unr  SampleTime=-1
  wires:
  gateway/1 -> workspace_input/1
  den_unr/1 -> gateway/1

== system kurtosis/kurtosis/absx_4th_im_ser ==
  load : Inport
  din_1 : Inport  Port=2
  din_2 : Inport  Port=3
  din_3 : Inport  Port=4
  din_4 : Inport  Port=5
  din_5 : Inport  Port=6
  din_6 : Inport  Port=7
  din_7 : Inport  Port=8
  din_8 : Inport  Port=9
  addr_counter : xbsIndex_r4/Counter  cnt_type=Free Running  cnt_to=Inf  operation=Up  start_count=0  cnt_by_val=1  arith_type=Unsigned  n_bits=4  bin_pt=0  load_pin=off  rst=on  en=off  explicit_period=on  period=1  dbl_ovrd=off  use_behavioral_HDL=off  implementation=Fabric  block_type=counter
  addr_del : xbsIndex_r4/Delay  rst=off  infoeditControl=Selection of Reset will increase slice count due to use of real FFs and instead of SRLs  en=off  latency=1  dbl_ovrd=off  reg_retiming=off  block_type=delay
  par_to_ser : Subsystem  AncestorBlock=casper_library_flow_control/parallel_to_serial_converter  mask(parallel_to_serial_converter){pin_width=672, sout_width=84}
      mask prompts: pin_width "Parallel Input Width"; sout_width "Serial Output Width"
      mask help:
      | This block takes as input a parallel bus of specified width.
      | When the load signal 'ld' is asserted, this data is broken into
      | pieces of width specified by the serial output width and
      | stored into different registers chained to form a shift register.
      | If the 'shift' input is subsequently asserted, the shift register
      | returns as output a new piece of data of width sout_width.  This data
      | is the next least significant piece of the original bus.  The converter
      | serializes SMALL ENDIAN.
      |
      | Note that the load operation automatically loads the least significant
      | bits into the register closest to the output, so the first 'shift'
      | assertion changes the data output from bits [sout_width-1:0] to
      | bits [2*sout_width-1:sout_width].
      mask init:
      | parallel_to_serial_converter_init(gcb, ...
      |     'pin_width', pin_width, ...
      |     'sout_width', sout_width);
  pin_concat : Subsystem
  pulse_ext : Subsystem
  reinterp : xbsIndex_r4/Reinterpret  force_arith_type=on  arith_type="Signed  (2's comp)"  force_bin_pt=on  bin_pt=68  block_type=reinterpret
  addr : Outport
  ser_data : Outport  Port=2
  valid : Outport  Port=3
  wires:
  load/1 -> addr_counter/1, par_to_ser/2(ld), pulse_ext/1(ld)
  pulse_ext/1(shift) -> par_to_ser/3(shift), valid/1  "shift"
  addr_del/1 -> addr/1
  addr_counter/1 -> addr_del/1
  reinterp/1 -> ser_data/1
  par_to_ser/1(sout) -> reinterp/1  "sout"
  pin_concat/1(out) -> par_to_ser/1(pin)
  din_8/1 -> pin_concat/8(in7)
  din_7/1 -> pin_concat/7(in6)
  din_6/1 -> pin_concat/6(in5)
  din_5/1 -> pin_concat/5(in4)
  din_4/1 -> pin_concat/4(in3)
  din_3/1 -> pin_concat/3(in2)
  din_2/1 -> pin_concat/2(in1)
  din_1/1 -> pin_concat/1(in0)

== system kurtosis/kurtosis/absx_sq_re_ser ==
  load : Inport
  din_1 : Inport  Port=2
  din_2 : Inport  Port=3
  din_3 : Inport  Port=4
  din_4 : Inport  Port=5
  din_5 : Inport  Port=6
  din_6 : Inport  Port=7
  din_7 : Inport  Port=8
  din_8 : Inport  Port=9
  addr_counter : xbsIndex_r4/Counter  cnt_type=Free Running  cnt_to=Inf  operation=Up  start_count=0  cnt_by_val=1  arith_type=Unsigned  n_bits=4  bin_pt=0  load_pin=off  rst=on  en=off  explicit_period=on  period=1  dbl_ovrd=off  use_behavioral_HDL=off  implementation=Fabric  block_type=counter
  addr_del : xbsIndex_r4/Delay  rst=off  infoeditControl=Selection of Reset will increase slice count due to use of real FFs and instead of SRLs  en=off  latency=1  dbl_ovrd=off  reg_retiming=off  block_type=delay
  par_to_ser : Subsystem  AncestorBlock=casper_library_flow_control/parallel_to_serial_converter  mask(parallel_to_serial_converter){pin_width=280, sout_width=35}
      mask prompts: pin_width "Parallel Input Width"; sout_width "Serial Output Width"
      mask help:
      | This block takes as input a parallel bus of specified width.
      | When the load signal 'ld' is asserted, this data is broken into
      | pieces of width specified by the serial output width and
      | stored into different registers chained to form a shift register.
      | If the 'shift' input is subsequently asserted, the shift register
      | returns as output a new piece of data of width sout_width.  This data
      | is the next least significant piece of the original bus.  The converter
      | serializes SMALL ENDIAN.
      |
      | Note that the load operation automatically loads the least significant
      | bits into the register closest to the output, so the first 'shift'
      | assertion changes the data output from bits [sout_width-1:0] to
      | bits [2*sout_width-1:sout_width].
      mask init:
      | parallel_to_serial_converter_init(gcb, ...
      |     'pin_width', pin_width, ...
      |     'sout_width', sout_width);
  pin_concat : Subsystem
  pulse_ext : Subsystem
  reinterp : xbsIndex_r4/Reinterpret  force_arith_type=on  arith_type="Signed  (2's comp)"  force_bin_pt=on  bin_pt=22  block_type=reinterpret
  addr : Outport
  ser_data : Outport  Port=2
  valid : Outport  Port=3
  wires:
  load/1 -> addr_counter/1, par_to_ser/2(ld), pulse_ext/1(ld)
  pulse_ext/1(shift) -> par_to_ser/3(shift), valid/1  "shift"
  addr_del/1 -> addr/1
  addr_counter/1 -> addr_del/1
  reinterp/1 -> ser_data/1
  par_to_ser/1(sout) -> reinterp/1  "sout"
  pin_concat/1(out) -> par_to_ser/1(pin)
  din_8/1 -> pin_concat/8(in7)
  din_7/1 -> pin_concat/7(in6)
  din_6/1 -> pin_concat/6(in5)
  din_5/1 -> pin_concat/5(in4)
  din_4/1 -> pin_concat/4(in3)
  din_3/1 -> pin_concat/3(in2)
  din_2/1 -> pin_concat/2(in1)
  din_1/1 -> pin_concat/1(in0)

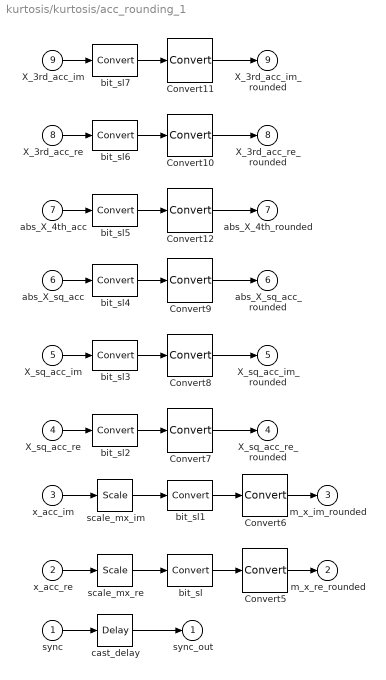
== system kurtosis/kurtosis/acc_rounding_1 ==
  sync : Inport
  x_acc_re : Inport  Port=2
  x_acc_im : Inport  Port=3
  X_sq_acc_re : Inport  Port=4
  X_sq_acc_im : Inport  Port=5
  abs_X_sq_acc : Inport  Port=6
  abs_X_4th_acc : Inport  Port=7
  X_3rd_acc_re : Inport  Port=8
  X_3rd_acc_im : Inport  Port=9
  Convert{7..11} (5 alike) : xbsIndex_r4/Convert  gui_display_data_type=Fixed-point  arith_type="Signed  (2's comp)"  n_bits=35  bin_pt=22  float_type=Single  exp_bits=8  fraction_bits=24  quantization="Round  (unbiased: +/- Inf)"  overflow=Saturate  en=off  latency=5  dbl_ovrd=off  pipeline=off  block_type=convert
  Convert12 : xbsIndex_r4/Convert  gui_display_data_type=Fixed-point  arith_type="Signed  (2's comp)"  n_bits=84  bin_pt=68  float_type=Single  exp_bits=8  fraction_bits=24  quantization="Round  (unbiased: +/- Inf)"  overflow=Saturate  en=off  latency=5  dbl_ovrd=off  pipeline=off  block_type=convert
  Convert5 : xbsIndex_r4/Convert  gui_display_data_type=Fixed-point  arith_type="Signed  (2's comp)"  n_bits=25  bin_pt=24  float_type=Single  exp_bits=8  fraction_bits=24  quantization="Round  (unbiased: +/- Inf)"  overflow=Saturate  en=off  latency=5  dbl_ovrd=off  pipeline=off  block_type=convert
  Convert6 : xbsIndex_r4/Convert  gui_display_data_type=Fixed-point  arith_type="Signed  (2's comp)"  n_bits=25  bin_pt=24  float_type=Single  exp_bits=8  fraction_bits=24  quantization="Round  (unbiased: +/- Inf)"  overflow=Saturate  en=off  latency=5  dbl_ovrd=off  pipeline=off  block_type=convert
  bit_sl : xbsIndex_r4/Convert  gui_display_data_type=Fixed-point  arith_type="Signed  (2's comp)"  n_bits=28  bin_pt=27  float_type=Single  exp_bits=8  fraction_bits=24  quantization=Truncate  overflow=Wrap  en=off  latency=0  dbl_ovrd=off  pipeline=off  block_type=convert
  bit_sl1 : xbsIndex_r4/Convert  gui_display_data_type=Fixed-point  arith_type="Signed  (2's comp)"  n_bits=28  bin_pt=27  float_type=Single  exp_bits=8  fraction_bits=24  quantization=Truncate  overflow=Wrap  en=off  latency=0  dbl_ovrd=off  pipeline=off  block_type=convert
  bit_sl2 : xbsIndex_r4/Convert  gui_display_data_type=Fixed-point  arith_type="Signed  (2's comp)"  n_bits=47  bin_pt=34  float_type=Single  exp_bits=8  fraction_bits=24  quantization=Truncate  overflow=Wrap  en=off  latency=0  dbl_ovrd=off  pipeline=off  block_type=convert
  bit_sl3 : xbsIndex_r4/Convert  gui_display_data_type=Fixed-point  arith_type="Signed  (2's comp)"  n_bits=47  bin_pt=34  float_type=Single  exp_bits=8  fraction_bits=24  quantization=Truncate  overflow=Wrap  en=off  latency=0  dbl_ovrd=off  pipeline=off  block_type=convert
  bit_sl4 : xbsIndex_r4/Convert  gui_display_data_type=Fixed-point  arith_type="Signed  (2's comp)"  n_bits=47  bin_pt=34  float_type=Single  exp_bits=8  fraction_bits=24  quantization=Truncate  overflow=Wrap  en=off  latency=0  dbl_ovrd=off  pipeline=off  block_type=convert
  bit_sl5 : xbsIndex_r4/Convert  gui_display_data_type=Fixed-point  arith_type="Signed  (2's comp)"  n_bits=84  bin_pt=68  float_type=Single  exp_bits=8  fraction_bits=24  quantization=Truncate  overflow=Wrap  en=off  latency=0  dbl_ovrd=off  pipeline=off  block_type=convert
  bit_sl6 : xbsIndex_r4/Convert  gui_display_data_type=Fixed-point  arith_type="Signed  (2's comp)"  n_bits=64  bin_pt=51  float_type=Single  exp_bits=8  fraction_bits=24  quantization=Truncate  overflow=Wrap  en=off  latency=0  dbl_ovrd=off  pipeline=off  block_type=convert
  bit_sl7 : xbsIndex_r4/Convert  gui_display_data_type=Fixed-point  arith_type="Signed  (2's comp)"  n_bits=64  bin_pt=51  float_type=Single  exp_bits=8  fraction_bits=24  quantization=Truncate  overflow=Wrap  en=off  latency=0  dbl_ovrd=off  pipeline=off  block_type=convert
  cast_delay : xbsIndex_r4/Delay  rst=off  infoeditControl=Selection of Reset will increase slice count due to use of real FFs and instead of SRLs  en=off  latency=5  dbl_ovrd=off  reg_retiming=off  block_type=delay
  scale_mx_im : xbsIndex_r4/Scale  scale_factor=-10  dbl_ovrd=off  block_type=scale
  scale_mx_re : xbsIndex_r4/Scale  scale_factor=-10  dbl_ovrd=off  block_type=scale
  sync_out : Outport
  m_x_re_rounded : Outport  Port=2
  m_x_im_rounded : Outport  Port=3
  X_sq_acc_re_rounded : Outport  Port=4
  X_sq_acc_im_rounded : Outport  Port=5
  abs_X_sq_acc_rounded : Outport  Port=6
  abs_X_4th_rounded : Outport  Port=7
  X_3rd_acc_re_rounded : Outport  Port=8
  X_3rd_acc_im_rounded : Outport  Port=9
  wires:
  cast_delay/1 -> sync_out/1
  sync/1 -> cast_delay/1
  Convert11/1 -> X_3rd_acc_im_rounded/1
  bit_sl7/1 -> Convert11/1
  Convert10/1 -> X_3rd_acc_re_rounded/1
  bit_sl6/1 -> Convert10/1
  Convert12/1 -> abs_X_4th_rounded/1
  bit_sl5/1 -> Convert12/1
  Convert9/1 -> abs_X_sq_acc_rounded/1
  bit_sl4/1 -> Convert9/1
  Convert8/1 -> X_sq_acc_im_rounded/1
  bit_sl3/1 -> Convert8/1
  Convert7/1 -> X_sq_acc_re_rounded/1
  bit_sl2/1 -> Convert7/1
  Convert6/1 -> m_x_im_rounded/1
  bit_sl1/1 -> Convert6/1
  Convert5/1 -> m_x_re_rounded/1
  bit_sl/1 -> Convert5/1
  X_3rd_acc_im/1 -> bit_sl7/1
  X_3rd_acc_re/1 -> bit_sl6/1
  abs_X_4th_acc/1 -> bit_sl5/1
  abs_X_sq_acc/1 -> bit_sl4/1
  X_sq_acc_im/1 -> bit_sl3/1
  X_sq_acc_re/1 -> bit_sl2/1
  scale_mx_im/1 -> bit_sl1/1
  scale_mx_re/1 -> bit_sl/1
  x_acc_im/1 -> scale_mx_im/1
  x_acc_re/1 -> scale_mx_re/1

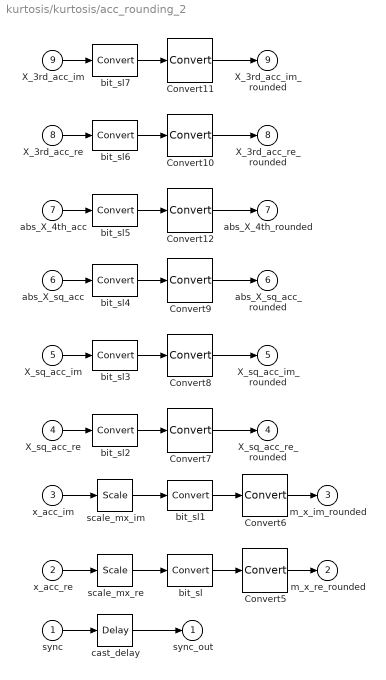
== system kurtosis/kurtosis/acc_rounding_2 ==
  sync : Inport
  x_acc_re : Inport  Port=2
  x_acc_im : Inport  Port=3
  X_sq_acc_re : Inport  Port=4
  X_sq_acc_im : Inport  Port=5
  abs_X_sq_acc : Inport  Port=6
  abs_X_4th_acc : Inport  Port=7
  X_3rd_acc_re : Inport  Port=8
  X_3rd_acc_im : Inport  Port=9
  Convert{7..11} (5 alike) : xbsIndex_r4/Convert  gui_display_data_type=Fixed-point  arith_type="Signed  (2's comp)"  n_bits=35  bin_pt=22  float_type=Single  exp_bits=8  fraction_bits=24  quantization="Round  (unbiased: +/- Inf)"  overflow=Saturate  en=off  latency=5  dbl_ovrd=off  pipeline=off  block_type=convert
  Convert12 : xbsIndex_r4/Convert  gui_display_data_type=Fixed-point  arith_type="Signed  (2's comp)"  n_bits=84  bin_pt=68  float_type=Single  exp_bits=8  fraction_bits=24  quantization="Round  (unbiased: +/- Inf)"  overflow=Saturate  en=off  latency=5  dbl_ovrd=off  pipeline=off  block_type=convert
  Convert5 : xbsIndex_r4/Convert  gui_display_data_type=Fixed-point  arith_type="Signed  (2's comp)"  n_bits=25  bin_pt=24  float_type=Single  exp_bits=8  fraction_bits=24  quantization="Round  (unbiased: +/- Inf)"  overflow=Saturate  en=off  latency=5  dbl_ovrd=off  pipeline=off  block_type=convert
  Convert6 : xbsIndex_r4/Convert  gui_display_data_type=Fixed-point  arith_type="Signed  (2's comp)"  n_bits=25  bin_pt=24  float_type=Single  exp_bits=8  fraction_bits=24  quantization="Round  (unbiased: +/- Inf)"  overflow=Saturate  en=off  latency=5  dbl_ovrd=off  pipeline=off  block_type=convert
  bit_sl : xbsIndex_r4/Convert  gui_display_data_type=Fixed-point  arith_type="Signed  (2's comp)"  n_bits=28  bin_pt=27  float_type=Single  exp_bits=8  fraction_bits=24  quantization=Truncate  overflow=Wrap  en=off  latency=0  dbl_ovrd=off  pipeline=off  block_type=convert
  bit_sl1 : xbsIndex_r4/Convert  gui_display_data_type=Fixed-point  arith_type="Signed  (2's comp)"  n_bits=28  bin_pt=27  float_type=Single  exp_bits=8  fraction_bits=24  quantization=Truncate  overflow=Wrap  en=off  latency=0  dbl_ovrd=off  pipeline=off  block_type=convert
  bit_sl2 : xbsIndex_r4/Convert  gui_display_data_type=Fixed-point  arith_type="Signed  (2's comp)"  n_bits=47  bin_pt=34  float_type=Single  exp_bits=8  fraction_bits=24  quantization=Truncate  overflow=Wrap  en=off  latency=0  dbl_ovrd=off  pipeline=off  block_type=convert
  bit_sl3 : xbsIndex_r4/Convert  gui_display_data_type=Fixed-point  arith_type="Signed  (2's comp)"  n_bits=47  bin_pt=34  float_type=Single  exp_bits=8  fraction_bits=24  quantization=Truncate  overflow=Wrap  en=off  latency=0  dbl_ovrd=off  pipeline=off  block_type=convert
  bit_sl4 : xbsIndex_r4/Convert  gui_display_data_type=Fixed-point  arith_type="Signed  (2's comp)"  n_bits=47  bin_pt=34  float_type=Single  exp_bits=8  fraction_bits=24  quantization=Truncate  overflow=Wrap  en=off  latency=0  dbl_ovrd=off  pipeline=off  block_type=convert
  bit_sl5 : xbsIndex_r4/Convert  gui_display_data_type=Fixed-point  arith_type="Signed  (2's comp)"  n_bits=84  bin_pt=68  float_type=Single  exp_bits=8  fraction_bits=24  quantization=Truncate  overflow=Wrap  en=off  latency=0  dbl_ovrd=off  pipeline=off  block_type=convert
  bit_sl6 : xbsIndex_r4/Convert  gui_display_data_type=Fixed-point  arith_type="Signed  (2's comp)"  n_bits=64  bin_pt=51  float_type=Single  exp_bits=8  fraction_bits=24  quantization=Truncate  overflow=Wrap  en=off  latency=0  dbl_ovrd=off  pipeline=off  block_type=convert
  bit_sl7 : xbsIndex_r4/Convert  gui_display_data_type=Fixed-point  arith_type="Signed  (2's comp)"  n_bits=64  bin_pt=51  float_type=Single  exp_bits=8  fraction_bits=24  quantization=Truncate  overflow=Wrap  en=off  latency=0  dbl_ovrd=off  pipeline=off  block_type=convert
  cast_delay : xbsIndex_r4/Delay  rst=off  infoeditControl=Selection of Reset will increase slice count due to use of real FFs and instead of SRLs  en=off  latency=5  dbl_ovrd=off  reg_retiming=off  block_type=delay
  scale_mx_im : xbsIndex_r4/Scale  scale_factor=-10  dbl_ovrd=off  block_type=scale
  scale_mx_re : xbsIndex_r4/Scale  scale_factor=-10  dbl_ovrd=off  block_type=scale
  sync_out : Outport
  m_x_re_rounded : Outport  Port=2
  m_x_im_rounded : Outport  Port=3
  X_sq_acc_re_rounded : Outport  Port=4
  X_sq_acc_im_rounded : Outport  Port=5
  abs_X_sq_acc_rounded : Outport  Port=6
  abs_X_4th_rounded : Outport  Port=7
  X_3rd_acc_re_rounded : Outport  Port=8
  X_3rd_acc_im_rounded : Outport  Port=9
  wires:
  cast_delay/1 -> sync_out/1
  sync/1 -> cast_delay/1
  Convert11/1 -> X_3rd_acc_im_rounded/1
  bit_sl7/1 -> Convert11/1
  Convert10/1 -> X_3rd_acc_re_rounded/1
  bit_sl6/1 -> Convert10/1
  Convert12/1 -> abs_X_4th_rounded/1
  bit_sl5/1 -> Convert12/1
  Convert9/1 -> abs_X_sq_acc_rounded/1
  bit_sl4/1 -> Convert9/1
  Convert8/1 -> X_sq_acc_im_rounded/1
  bit_sl3/1 -> Convert8/1
  Convert7/1 -> X_sq_acc_re_rounded/1
  bit_sl2/1 -> Convert7/1
  Convert6/1 -> m_x_im_rounded/1
  bit_sl1/1 -> Convert6/1
  Convert5/1 -> m_x_re_rounded/1
  bit_sl/1 -> Convert5/1
  X_3rd_acc_im/1 -> bit_sl7/1
  X_3rd_acc_re/1 -> bit_sl6/1
  abs_X_4th_acc/1 -> bit_sl5/1
  abs_X_sq_acc/1 -> bit_sl4/1
  X_sq_acc_im/1 -> bit_sl3/1
  X_sq_acc_re/1 -> bit_sl2/1
  scale_mx_im/1 -> bit_sl1/1
  scale_mx_re/1 -> bit_sl/1
  x_acc_im/1 -> scale_mx_im/1
  x_acc_re/1 -> scale_mx_re/1
